simulink model "v00_0A_0E"  (R2022b)
settings: Solver=FixedStepDiscrete  StartTime=0.0  StopTime=8000  FixedStep=SampleTime  MaxStep=Contactors_StepTime_msec  RelTol=1e-3  EnableMultiTasking=on
undefined symbols (not defined in the file): A_to_mA, BalancingTempGroup, canChannel, CapacityFactor, CC_Inputs, CellSOC, ChargeState, ContactorsFlags, DiscIntNeverNeededParam, gEN_Contactors_StepTime_msec, Ion, isDynamicCurrentEn, Lithium, maxAllowedImbalance, nCells_parallel, nCells_series, nCellTempGrps, PermanentFailRecoveryTrigger, ProtectionFlags, RBal_ohm, SampleTime, sigbuilder_block, StLineEq_varA, StLineEq_varB, TempSelectForDCL, Thresholds, V_to_mV
libraries: simulink x32, spsIdealSwitchLib x21, spsBatteryLib x20, spsSeriesRLCBranchLib x20, spsVoltageMeasurementLib x20, canmsglib x4, canlib x3, dspstat3 x2, spspowerguiLib x2, spsControlledCurrentSourceLib x1, spsCurrentMeasurementLib x1
(part 2 of 7)

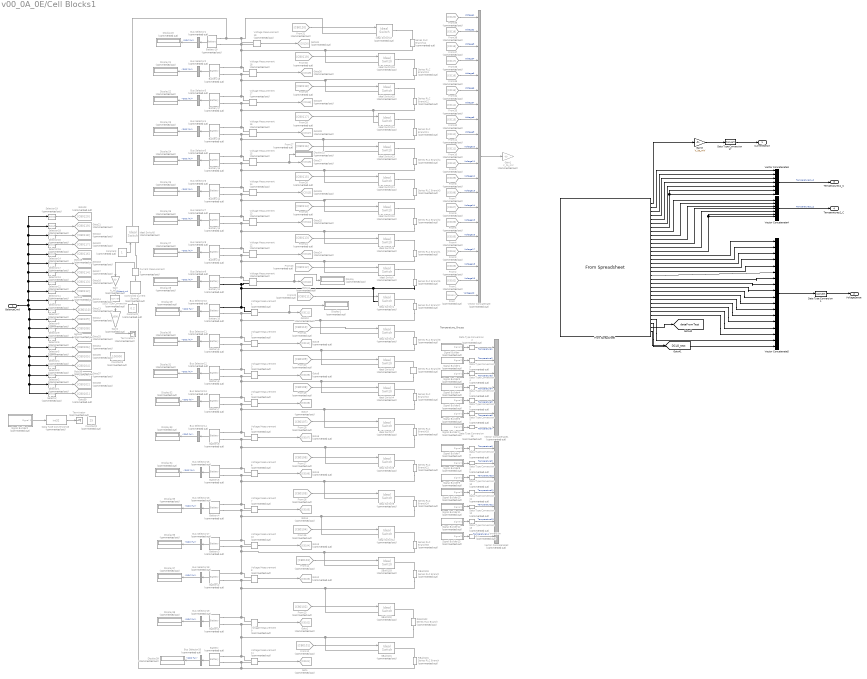
== system v00_0A_0E/Cell Blocks1 ==
  note: Temperature_Groups
  BalanceCmd : Inport
  Battery : spsBatteryLib/Battery  Commented=on  BatType=Lithium-Ion  ShowTempParam=off  ThermalPreset=no  ShowAgeParam=off  NomV=3.6  NomQ=CellCapacity_mAh  SOC=CellSOC(1)  Batt_Tr=30  PresetModel=on  MaxQ=4  MinV=2.7  FullV=4.1904  Dis_rate=1.7391  R=0.009  Normal_OP=3.6174  expZone="[3.8894     0.19652]"  current=[6.5 13 32.5]  Units=Time  Tci=20  NomT=20  T2=-30  MaxQ2=4.8  FullV2=7.1  Normal_OP2=5.655  expZone2="[6.58           1]"  Rca=0.6  ti=2000  Dp=0  Neq0=0  Tsim=1e6  Ta1=25  Qeol=5.4*0.9  Reol=0.013333*1.2  Char_age=[2.3478, 3]  Dis_age=[2.3478, 10]  N1=1500  N2=10500  N3=1000  N4=1400  Ta2=45  N5=950
  Battery1 : spsBatteryLib/Battery  Commented=on  BatType=Lithium-Ion  ShowTempParam=off  ThermalPreset=no  ShowAgeParam=off  NomV=3.6  NomQ=CellCapacity_mAh  SOC=CellSOC(2)  Batt_Tr=30  PresetModel=on  MaxQ=4  MinV=2.7  FullV=4.1904  Dis_rate=1.7391  R=0.009  Normal_OP=3.6174  expZone="[3.8894     0.19652]"  current=[6.5 13 32.5]  Units=Time  Tci=20  NomT=20  T2=-30  MaxQ2=4.8  FullV2=7.1  Normal_OP2=5.655  expZone2="[6.58           1]"  Rca=0.6  ti=2000  Dp=0  Neq0=0  Tsim=1e6  Ta1=25  Qeol=5.4*0.9  Reol=0.013333*1.2  Char_age=[2.3478, 3]  Dis_age=[2.3478, 10]  N1=1500  N2=10500  N3=1000  N4=1400  Ta2=45  N5=950
  Battery10 : spsBatteryLib/Battery  Commented=on  BatType=Lithium-Ion  ShowTempParam=off  ThermalPreset=no  ShowAgeParam=off  NomV=3.6  NomQ=CellCapacity_mAh  SOC=CellSOC(10)  Batt_Tr=30  PresetModel=on  MaxQ=4  MinV=2.7  FullV=4.1904  Dis_rate=1.7391  R=0.009  Normal_OP=3.6174  expZone="[3.8894     0.19652]"  current=[6.5 13 32.5]  Units=Time  Tci=20  NomT=20  T2=-30  MaxQ2=4.8  FullV2=7.1  Normal_OP2=5.655  expZone2="[6.58           1]"  Rca=0.6  ti=2000  Dp=0  Neq0=0  Tsim=1e6  Ta1=25  Qeol=5.4*0.9  Reol=0.013333*1.2  Char_age=[2.3478, 3]  Dis_age=[2.3478, 10]  N1=1500  N2=10500  N3=1000  N4=1400  Ta2=45  N5=950
  Battery{11..19} (9 alike) : spsBatteryLib/Battery  Commented=on  BatType=Lithium-Ion  ShowTempParam=off  ThermalPreset=no  ShowAgeParam=off  NomV=3.6  NomQ=CellCapacity_mAh  SOC=CellSOC(11)  Batt_Tr=30  PresetModel=on  MaxQ=4  MinV=2.7  FullV=4.1904  Dis_rate=1.7391  R=0.009  Normal_OP=3.6174  expZone="[3.8894     0.19652]"  current=[6.5 13 32.5]  Units=Time  Tci=20  NomT=20  T2=-30  MaxQ2=4.8  FullV2=7.1  Normal_OP2=5.655  expZone2="[6.58           1]"  Rca=0.6  ti=2000  Dp=0  Neq0=0  Tsim=1e6  Ta1=25  Qeol=5.4*0.9  Reol=0.013333*1.2  Char_age=[2.3478, 3]  Dis_age=[2.3478, 10]  N1=1500  N2=10500  N3=1000  N4=1400  Ta2=45  N5=950
  Battery2 : spsBatteryLib/Battery  Commented=on  BatType=Lithium-Ion  ShowTempParam=off  ThermalPreset=no  ShowAgeParam=off  NomV=3.6  NomQ=CellCapacity_mAh  SOC=CellSOC(3)  Batt_Tr=30  PresetModel=on  MaxQ=4  MinV=2.7  FullV=4.1904  Dis_rate=1.7391  R=0.009  Normal_OP=3.6174  expZone="[3.8894     0.19652]"  current=[6.5 13 32.5]  Units=Time  Tci=20  NomT=20  T2=-30  MaxQ2=4.8  FullV2=7.1  Normal_OP2=5.655  expZone2="[6.58           1]"  Rca=0.6  ti=2000  Dp=0  Neq0=0  Tsim=1e6  Ta1=25  Qeol=5.4*0.9  Reol=0.013333*1.2  Char_age=[2.3478, 3]  Dis_age=[2.3478, 10]  N1=1500  N2=10500  N3=1000  N4=1400  Ta2=45  N5=950
  Battery3 : spsBatteryLib/Battery  Commented=on  BatType=Lithium-Ion  ShowTempParam=off  ThermalPreset=no  ShowAgeParam=off  NomV=3.6  NomQ=CellCapacity_mAh  SOC=CellSOC(4)  Batt_Tr=30  PresetModel=on  MaxQ=4  MinV=2.7  FullV=4.1904  Dis_rate=1.7391  R=0.009  Normal_OP=3.6174  expZone="[3.8894     0.19652]"  current=[6.5 13 32.5]  Units=Time  Tci=20  NomT=20  T2=-30  MaxQ2=4.8  FullV2=7.1  Normal_OP2=5.655  expZone2="[6.58           1]"  Rca=0.6  ti=2000  Dp=0  Neq0=0  Tsim=1e6  Ta1=25  Qeol=5.4*0.9  Reol=0.013333*1.2  Char_age=[2.3478, 3]  Dis_age=[2.3478, 10]  N1=1500  N2=10500  N3=1000  N4=1400  Ta2=45  N5=950
  Battery4 : spsBatteryLib/Battery  Commented=on  BatType=Lithium-Ion  ShowTempParam=off  ThermalPreset=no  ShowAgeParam=off  NomV=3.6  NomQ=CellCapacity_mAh  SOC=CellSOC(5)  Batt_Tr=30  PresetModel=on  MaxQ=4  MinV=2.7  FullV=4.1904  Dis_rate=1.7391  R=0.009  Normal_OP=3.6174  expZone="[3.8894     0.19652]"  current=[6.5 13 32.5]  Units=Time  Tci=20  NomT=20  T2=-30  MaxQ2=4.8  FullV2=7.1  Normal_OP2=5.655  expZone2="[6.58           1]"  Rca=0.6  ti=2000  Dp=0  Neq0=0  Tsim=1e6  Ta1=25  Qeol=5.4*0.9  Reol=0.013333*1.2  Char_age=[2.3478, 3]  Dis_age=[2.3478, 10]  N1=1500  N2=10500  N3=1000  N4=1400  Ta2=45  N5=950
  Battery5 : spsBatteryLib/Battery  Commented=on  BatType=Lithium-Ion  ShowTempParam=off  ThermalPreset=no  ShowAgeParam=off  NomV=3.6  NomQ=CellCapacity_mAh  SOC=CellSOC(6)  Batt_Tr=30  PresetModel=on  MaxQ=4  MinV=2.7  FullV=4.1904  Dis_rate=1.7391  R=0.009  Normal_OP=3.6174  expZone="[3.8894     0.19652]"  current=[6.5 13 32.5]  Units=Time  Tci=20  NomT=20  T2=-30  MaxQ2=4.8  FullV2=7.1  Normal_OP2=5.655  expZone2="[6.58           1]"  Rca=0.6  ti=2000  Dp=0  Neq0=0  Tsim=1e6  Ta1=25  Qeol=5.4*0.9  Reol=0.013333*1.2  Char_age=[2.3478, 3]  Dis_age=[2.3478, 10]  N1=1500  N2=10500  N3=1000  N4=1400  Ta2=45  N5=950
  Battery6 : spsBatteryLib/Battery  Commented=on  BatType=Lithium-Ion  ShowTempParam=off  ThermalPreset=no  ShowAgeParam=off  NomV=3.6  NomQ=CellCapacity_mAh  SOC=CellSOC(7)  Batt_Tr=30  PresetModel=on  MaxQ=4  MinV=2.7  FullV=4.1904  Dis_rate=1.7391  R=0.009  Normal_OP=3.6174  expZone="[3.8894     0.19652]"  current=[6.5 13 32.5]  Units=Time  Tci=20  NomT=20  T2=-30  MaxQ2=4.8  FullV2=7.1  Normal_OP2=5.655  expZone2="[6.58           1]"  Rca=0.6  ti=2000  Dp=0  Neq0=0  Tsim=1e6  Ta1=25  Qeol=5.4*0.9  Reol=0.013333*1.2  Char_age=[2.3478, 3]  Dis_age=[2.3478, 10]  N1=1500  N2=10500  N3=1000  N4=1400  Ta2=45  N5=950
  Battery7 : spsBatteryLib/Battery  Commented=on  BatType=Lithium-Ion  ShowTempParam=off  ThermalPreset=no  ShowAgeParam=off  NomV=3.6  NomQ=CellCapacity_mAh  SOC=CellSOC(8)  Batt_Tr=30  PresetModel=on  MaxQ=4  MinV=2.7  FullV=4.1904  Dis_rate=1.7391  R=0.009  Normal_OP=3.6174  expZone="[3.8894     0.19652]"  current=[6.5 13 32.5]  Units=Time  Tci=20  NomT=20  T2=-30  MaxQ2=4.8  FullV2=7.1  Normal_OP2=5.655  expZone2="[6.58           1]"  Rca=0.6  ti=2000  Dp=0  Neq0=0  Tsim=1e6  Ta1=25  Qeol=5.4*0.9  Reol=0.013333*1.2  Char_age=[2.3478, 3]  Dis_age=[2.3478, 10]  N1=1500  N2=10500  N3=1000  N4=1400  Ta2=45  N5=950
  Battery8 : spsBatteryLib/Battery  Commented=on  BatType=Lithium-Ion  ShowTempParam=off  ThermalPreset=no  ShowAgeParam=off  NomV=3.6  NomQ=CellCapacity_mAh  SOC=CellSOC(8)  Batt_Tr=30  PresetModel=on  MaxQ=4  MinV=2.7  FullV=4.1904  Dis_rate=1.7391  R=0.009  Normal_OP=3.6174  expZone="[3.8894     0.19652]"  current=[6.5 13 32.5]  Units=Time  Tci=20  NomT=20  T2=-30  MaxQ2=4.8  FullV2=7.1  Normal_OP2=5.655  expZone2="[6.58           1]"  Rca=0.6  ti=2000  Dp=0  Neq0=0  Tsim=1e6  Ta1=25  Qeol=5.4*0.9  Reol=0.013333*1.2  Char_age=[2.3478, 3]  Dis_age=[2.3478, 10]  N1=1500  N2=10500  N3=1000  N4=1400  Ta2=45  N5=950
  Battery9 : spsBatteryLib/Battery  Commented=on  BatType=Lithium-Ion  ShowTempParam=off  ThermalPreset=no  ShowAgeParam=off  NomV=3.6  NomQ=CellCapacity_mAh  SOC=CellSOC(9)  Batt_Tr=30  PresetModel=on  MaxQ=4  MinV=2.7  FullV=4.1904  Dis_rate=1.7391  R=0.009  Normal_OP=3.6174  expZone="[3.8894     0.19652]"  current=[6.5 13 32.5]  Units=Time  Tci=20  NomT=20  T2=-30  MaxQ2=4.8  FullV2=7.1  Normal_OP2=5.655  expZone2="[6.58           1]"  Rca=0.6  ti=2000  Dp=0  Neq0=0  Tsim=1e6  Ta1=25  Qeol=5.4*0.9  Reol=0.013333*1.2  Char_age=[2.3478, 3]  Dis_age=[2.3478, 10]  N1=1500  N2=10500  N3=1000  N4=1400  Ta2=45  N5=950
  Bus Selector{1..20} (20 alike) : BusSelector  Commented=on  OutputSignals=SOC (%)
  Constant : Constant  Commented=on
  Constant1 : Constant  Commented=on  Value=0.2
  Constant2 : Constant  Commented=on  Value=25  OutDataTypeStr=int8
  Constant3 : Constant  Commented=on  Value=100000  OutDataTypeStr=int32
  Controlled Current Source1 : spsControlledCurrentSourceLib/Controlled Current Source  Commented=on  Initialize=on  Source_Type=DC  Amplitude=0.5  Phase=0  Frequency=0  Measurements=None
  Current Measurement1 : spsCurrentMeasurementLib/Current Measurement  Commented=on  PhasorSimulation=off  OutputType=Complex  PSBequivalent=0
  Data Type Conversion : DataTypeConversion  Commented=on  SaturateOnIntegerOverflow=off  RndMeth=Floor
  Data Type Conversion1 : DataTypeConversion  SaturateOnIntegerOverflow=off  RndMeth=Floor
  Data Type Conversion{2..15} (14 alike) : DataTypeConversion  Commented=on  OutDataTypeStr=int16  SaturateOnIntegerOverflow=off  RndMeth=Floor
  Data Type Conversion16 : DataTypeConversion  Commented=on  OutDataTypeStr=int32  SaturateOnIntegerOverflow=off  RndMeth=Floor
  Data Type Conversion17 : DataTypeConversion  SaturateOnIntegerOverflow=off  RndMeth=Floor
  Display{,1,15,20..39} (23 alike) : Display  Commented=on
  From : From  Commented=on  GotoTag=C0101
  From Spreadsheet : FromSpreadsheet  FileName=latchcheckcharge.xlsx
  From1 : From  Commented=on  GotoTag=C0102
  From10 : From  Commented=on  GotoTag=C0111
  From11 : From  Commented=on  GotoTag=C0112
  From12 : From  Commented=on  GotoTag=CB0101
  From13 : From  Commented=on  GotoTag=CB0102
  From14 : From  Commented=on  GotoTag=CB0103
  From15 : From  Commented=on  GotoTag=CB0104
  From16 : From  Commented=on  GotoTag=CB0105
  From17 : From  Commented=on  GotoTag=CB0106
  From18 : From  Commented=on  GotoTag=CB0107
  From19 : From  Commented=on  GotoTag=CB0108
  From2 : From  Commented=on  GotoTag=C0103
  From20 : From  Commented=on  GotoTag=CB0109
  From21 : From  Commented=on  GotoTag=CB0110
  From22 : From  Commented=on  GotoTag=CB0111
  From23 : From  Commented=on  GotoTag=CB0112
  From24 : From  Commented=on  GotoTag=CB0113
  From25 : From  Commented=on  GotoTag=CB0114
  From26 : From  Commented=on  GotoTag=CB0115
  From27 : From  Commented=on  GotoTag=CB0116
  From28 : From  Commented=on  GotoTag=CB0117
  From29 : From  Commented=on  GotoTag=CB0118
  From3 : From  Commented=on  GotoTag=C0104
  From30 : From  Commented=on  GotoTag=CB0119
  From31 : From  Commented=on  GotoTag=CB0120
  From32 : From  Commented=on  GotoTag=C0113
  From33 : From  Commented=on  GotoTag=C0114
  From34 : From  Commented=on  GotoTag=C0115
  From35 : From  Commented=on  GotoTag=C0116
  From36 : From  Commented=on  GotoTag=C0117
  From37 : From  Commented=on  GotoTag=C0118
  From38 : From  Commented=on  GotoTag=C0119
  From39 : From  Commented=on  GotoTag=C0120
  From4 : From  Commented=on  GotoTag=C0105
  From5 : From  Commented=on  GotoTag=C0106
  From6 : From  Commented=on  GotoTag=C0107
  From7 : From  Commented=on  GotoTag=C0108
  From8 : From  Commented=on  GotoTag=C0109
  From9 : From  Commented=on  GotoTag=C0110
  Gain : Gain  Commented=on  Gain=A_to_mA
  Gain1 : Gain  Commented=on  Gain=V_to_mV
  Gain2 : Gain  Commented=on  Gain=1000  OutDataTypeStr=int32
  Gain3 : Gain  Gain=V_to_mV
  Goto : Goto  Commented=on  GotoTag=C0101
  Goto1 : Goto  Commented=on  GotoTag=C0102
  Goto10 : Goto  Commented=on  GotoTag=C0111
  Goto11 : Goto  Commented=on  GotoTag=C0112
  Goto12 : Goto  Commented=on  GotoTag=CB0109
  Goto13 : Goto  Commented=on  GotoTag=CB0110
  Goto14 : Goto  Commented=on  GotoTag=CB0111
  Goto15 : Goto  Commented=on  GotoTag=CB0112
  Goto16 : Goto  Commented=on  GotoTag=CB0113
  Goto17 : Goto  Commented=on  GotoTag=CB0114
  Goto18 : Goto  Commented=on  GotoTag=CB0115
  Goto19 : Goto  Commented=on  GotoTag=CB0116
  Goto2 : Goto  Commented=on  GotoTag=C0103
  Goto20 : Goto  Commented=on  GotoTag=CB0117
  Goto21 : Goto  Commented=on  GotoTag=CB0119
  Goto22 : Goto  Commented=on  GotoTag=CB0118
  Goto23 : Goto  Commented=on  GotoTag=CB0120
  Goto24 : Goto  Commented=on  GotoTag=C0113
  Goto25 : Goto  Commented=on  GotoTag=C0114
  Goto26 : Goto  Commented=on  GotoTag=C0115
  Goto27 : Goto  Commented=on  GotoTag=C0116
  Goto28 : Goto  Commented=on  GotoTag=C0117
  Goto29 : Goto  Commented=on  GotoTag=C0118
  Goto3 : Goto  Commented=on  GotoTag=C0104
  Goto30 : Goto  Commented=on  GotoTag=C0119
  Goto31 : Goto  Commented=on  GotoTag=C0120
  Goto32 : Goto  Commented=on  GotoTag=CB0108
  Goto33 : Goto  Commented=on  GotoTag=CB0107
  Goto34 : Goto  Commented=on  GotoTag=CB0106
  Goto35 : Goto  Commented=on  GotoTag=CB0105
  Goto36 : Goto  Commented=on  GotoTag=CB0104
  Goto37 : Goto  Commented=on  GotoTag=CB0103
  Goto38 : Goto  Commented=on  GotoTag=CB0102
  Goto39 : Goto  Commented=on  GotoTag=CB0101
  Goto4 : Goto  Commented=on  GotoTag=C0105
  Goto5 : Goto  Commented=on  GotoTag=C0106
  Goto6 : Goto  Commented=on  GotoTag=C0107
  Goto7 : Goto  Commented=on  GotoTag=C0108
  Goto8 : Goto  Commented=on  GotoTag=C0109
  Goto9 : Goto  Commented=on  GotoTag=C0110
  Ideal Switch{,1..17} (18 alike) : spsIdealSwitchLib/Ideal Switch  Commented=on  Ron=0.1  Lon=0  IC=0  Rs=1e5  Cs=inf  Measurements=off
  RBal0101 : spsSeriesRLCBranchLib/Series RLC Branch  Commented=on  LConnTagsString=__new0  RConnTagsString=__new0  BranchType=R  Resistance=RBal_ohm  Inductance=0  SetiL0=off  InitialCurrent=0  Capacitance=1e-20  Setx0=off  InitialVoltage=0  Measurements=None
  RBal0102 : spsSeriesRLCBranchLib/Series RLC Branch  Commented=on  LConnTagsString=__new0  RConnTagsString=__new0  BranchType=R  Resistance=RBal_ohm  Inductance=0  SetiL0=off  InitialCurrent=0  Capacitance=1e-20  Setx0=off  InitialVoltage=0  Measurements=None
  RBal0103 : spsSeriesRLCBranchLib/Series RLC Branch  Commented=on  LConnTagsString=__new0  RConnTagsString=__new0  BranchType=R  Resistance=RBal_ohm  Inductance=0  SetiL0=off  InitialCurrent=0  Capacitance=1e-20  Setx0=off  InitialVoltage=0  Measurements=None
  SBal0101 : spsIdealSwitchLib/Ideal Switch  Commented=on  Ron=0.1  Lon=0  IC=0  Rs=1e5  Cs=inf  Measurements=off
  SBal0102 : spsIdealSwitchLib/Ideal Switch  Commented=on  Ron=0.1  Lon=0  IC=0  Rs=1e5  Cs=inf  Measurements=off
  SBal0103 : spsIdealSwitchLib/Ideal Switch  Commented=on  Ron=0.1  Lon=0  IC=0  Rs=1e5  Cs=inf  Measurements=off
  Selector : Selector  Commented=on  IndexMode=Zero-based  InputPortWidth=20  IndexOptions=Index vector (dialog)  Indices=[19]  OutputSizes=1
  Selector1 : Selector  Commented=on  IndexMode=Zero-based  InputPortWidth=20  IndexOptions=Index vector (dialog)  Indices=[18]  OutputSizes=1
  Selector10 : Selector  Commented=on  IndexMode=Zero-based  InputPortWidth=20  IndexOptions=Index vector (dialog)  Indices=[9]  OutputSizes=1
  Selector11 : Selector  Commented=on  IndexMode=Zero-based  InputPortWidth=20  IndexOptions=Index vector (dialog)  Indices=[8]  OutputSizes=1
  Selector12 : Selector  Commented=on  IndexMode=Zero-based  InputPortWidth=20  IndexOptions=Index vector (dialog)  Indices=[7]  OutputSizes=1
  Selector13 : Selector  Commented=on  IndexMode=Zero-based  InputPortWidth=20  IndexOptions=Index vector (dialog)  Indices=[6]  OutputSizes=1
  Selector14 : Selector  Commented=on  IndexMode=Zero-based  InputPortWidth=20  IndexOptions=Index vector (dialog)  Indices=[4]  OutputSizes=1
  Selector15 : Selector  Commented=on  IndexMode=Zero-based  InputPortWidth=20  IndexOptions=Index vector (dialog)  Indices=[2]  OutputSizes=1
  Selector16 : Selector  Commented=on  IndexMode=Zero-based  InputPortWidth=20  IndexOptions=Index vector (dialog)  Indices=[3]  OutputSizes=1
  Selector17 : Selector  Commented=on  IndexMode=Zero-based  InputPortWidth=20  IndexOptions=Index vector (dialog)  Indices=[5]  OutputSizes=1
  Selector18 : Selector  Commented=on  IndexMode=Zero-based  InputPortWidth=20  IndexOptions=Index vector (dialog)  Indices=[1]  OutputSizes=1
  Selector19 : Selector  Commented=on  IndexMode=Zero-based  InputPortWidth=20  IndexOptions=Index vector (dialog)  Indices=[0]  OutputSizes=1
  Selector2 : Selector  Commented=on  IndexMode=Zero-based  InputPortWidth=20  IndexOptions=Index vector (dialog)  Indices=[17]  OutputSizes=1
  Selector3 : Selector  Commented=on  IndexMode=Zero-based  InputPortWidth=20  IndexOptions=Index vector (dialog)  Indices=[16]  OutputSizes=1
  Selector4 : Selector  Commented=on  IndexMode=Zero-based  InputPortWidth=20  IndexOptions=Index vector (dialog)  Indices=[15]  OutputSizes=1
  Selector5 : Selector  Commented=on  IndexMode=Zero-based  InputPortWidth=20  IndexOptions=Index vector (dialog)  Indices=[14]  OutputSizes=1
  Selector6 : Selector  Commented=on  IndexMode=Zero-based  InputPortWidth=20  IndexOptions=Index vector (dialog)  Indices=[13]  OutputSizes=1
  Selector7 : Selector  Commented=on  IndexMode=Zero-based  InputPortWidth=20  IndexOptions=Index vector (dialog)  Indices=[10]  OutputSizes=1
  Selector8 : Selector  Commented=on  IndexMode=Zero-based  InputPortWidth=20  IndexOptions=Index vector (dialog)  Indices=[11]  OutputSizes=1
  Selector9 : Selector  Commented=on  IndexMode=Zero-based  InputPortWidth=20  IndexOptions=Index vector (dialog)  Indices=[12]  OutputSizes=1
  Series RLC Branch{1..5,7..14,18,21,24,33} (17 alike) : spsSeriesRLCBranchLib/Series RLC Branch  Commented=on  LConnTagsString=__new0  RConnTagsString=__new0  BranchType=R  Resistance=RBal_ohm  Inductance=0  SetiL0=off  InitialCurrent=0  Capacitance=1e-20  Setx0=off  InitialVoltage=0  Measurements=None
  Signal Builder : Subsystem  Tag=STV Subsys  Commented=on  LoadFcn=sigbuilder_block('load');  StartFcn=sigbuilder_block('start');  StopFcn=sigbuilder_block('stop');  ClipboardFcn=sigbuilder_block('clipboard');  mask(Sigbuilder block){tuvar=[0:10]}
      mask help: Simulink:masks:SigbuilderBlock_MD
      mask init:
      | if ~strcmp(get_param(bdroot(gcbh),'SimulationStatus'),'stopped') tuvar = sigbuilder_block('maskInit'); end
      settings: CopyFcn=sigbuilder_block('copy');  DeleteFcn=sigbuilder_block('delete');  ModelCloseFcn=sigbuilder_block('modelClose');  PreSaveFcn=sigbuilder_block('preSave');  PauseFcn=sigbuilder_block('pause');  ContinueFcn=sigbuilder_block('continue');  NameChangeFcn=sigbuilder_block('namechange');  OpenFcn=sigbuilder_block('open',[5.4 30 1141.2 522.6 ]);  CloseFcn=sigbuilder_block('close');
      mask Display: plot(0, 0, 100, 100,[2, 2, 32, 32, 2], [68, 8, 8, 68, 68],[32, 2], [38, 38], [32, 19, 2],[53, 60, 44], [32, 17, 17, 2],[16, 16, 31, 31]);txt = getActiveGroup(gcbh);text(2, 100, txt,'verticalAlignment', 'top');
  Signal Builder1 : Subsystem  Tag=STV Subsys  Commented=on  LoadFcn=sigbuilder_block('load');  StartFcn=sigbuilder_block('start');  StopFcn=sigbuilder_block('stop');  ClipboardFcn=sigbuilder_block('clipboard');  mask(Sigbuilder block){tuvar=[0:10]}
      mask help: Simulink:masks:SigbuilderBlock_MD
      mask init:
      | if ~strcmp(get_param(bdroot(gcbh),'SimulationStatus'),'stopped') tuvar = sigbuilder_block('maskInit'); end
      settings: CopyFcn=sigbuilder_block('copy');  DeleteFcn=sigbuilder_block('delete');  ModelCloseFcn=sigbuilder_block('modelClose');  PreSaveFcn=sigbuilder_block('preSave');  PauseFcn=sigbuilder_block('pause');  ContinueFcn=sigbuilder_block('continue');  NameChangeFcn=sigbuilder_block('namechange');  OpenFcn=sigbuilder_block('open',[5.4 30 1141.2 522.6 ]);  CloseFcn=sigbuilder_block('close');
      mask Display: plot(0, 0, 100, 100,[2, 2, 32, 32, 2], [68, 8, 8, 68, 68],[32, 2], [38, 38], [32, 19, 2],[53, 60, 44], [32, 17, 17, 2],[16, 16, 31, 31]);txt = getActiveGroup(gcbh);text(2, 100, txt,'verticalAlignment', 'top');
  Signal Builder10 : Subsystem  Tag=STV Subsys  Commented=on  LoadFcn=sigbuilder_block('load');  StartFcn=sigbuilder_block('start');  StopFcn=sigbuilder_block('stop');  ClipboardFcn=sigbuilder_block('clipboard');  mask(Sigbuilder block){tuvar=[0:10]}
      mask help: Simulink:masks:SigbuilderBlock_MD
      mask init:
      | if ~strcmp(get_param(bdroot(gcbh),'SimulationStatus'),'stopped') tuvar = sigbuilder_block('maskInit'); end
      settings: CopyFcn=sigbuilder_block('copy');  DeleteFcn=sigbuilder_block('delete');  ModelCloseFcn=sigbuilder_block('modelClose');  PreSaveFcn=sigbuilder_block('preSave');  PauseFcn=sigbuilder_block('pause');  ContinueFcn=sigbuilder_block('continue');  NameChangeFcn=sigbuilder_block('namechange');  OpenFcn=sigbuilder_block('open',[0 30 1152 561.6 ]);  CloseFcn=sigbuilder_block('close');
      mask Display: plot(0, 0, 100, 100,[2, 2, 32, 32, 2], [68, 8, 8, 68, 68],[32, 2], [38, 38], [32, 19, 2],[53, 60, 44], [32, 17, 17, 2],[16, 16, 31, 31]);txt = getActiveGroup(gcbh);text(2, 100, txt,'verticalAlignment', 'top');
  Signal Builder11 : Subsystem  Tag=STV Subsys  Commented=on  LoadFcn=sigbuilder_block('load');  StartFcn=sigbuilder_block('start');  StopFcn=sigbuilder_block('stop');  ClipboardFcn=sigbuilder_block('clipboard');  mask(Sigbuilder block){tuvar=[0:10]}
      mask help: Simulink:masks:SigbuilderBlock_MD
      mask init:
      | if ~strcmp(get_param(bdroot(gcbh),'SimulationStatus'),'stopped') tuvar = sigbuilder_block('maskInit'); end
      settings: CopyFcn=sigbuilder_block('copy');  DeleteFcn=sigbuilder_block('delete');  ModelCloseFcn=sigbuilder_block('modelClose');  PreSaveFcn=sigbuilder_block('preSave');  PauseFcn=sigbuilder_block('pause');  ContinueFcn=sigbuilder_block('continue');  NameChangeFcn=sigbuilder_block('namechange');  OpenFcn=sigbuilder_block('open',[0 30 1152 561.6 ]);  CloseFcn=sigbuilder_block('close');
      mask Display: plot(0, 0, 100, 100,[2, 2, 32, 32, 2], [68, 8, 8, 68, 68],[32, 2], [38, 38], [32, 19, 2],[53, 60, 44], [32, 17, 17, 2],[16, 16, 31, 31]);txt = getActiveGroup(gcbh);text(2, 100, txt,'verticalAlignment', 'top');
  Signal Builder12 : Subsystem  Tag=STV Subsys  Commented=on  LoadFcn=sigbuilder_block('load');  StartFcn=sigbuilder_block('start');  StopFcn=sigbuilder_block('stop');  ClipboardFcn=sigbuilder_block('clipboard');  mask(Sigbuilder block){tuvar=[0:10]}
      mask help: Simulink:masks:SigbuilderBlock_MD
      mask init:
      | if ~strcmp(get_param(bdroot(gcbh),'SimulationStatus'),'stopped') tuvar = sigbuilder_block('maskInit'); end
      settings: CopyFcn=sigbuilder_block('copy');  DeleteFcn=sigbuilder_block('delete');  ModelCloseFcn=sigbuilder_block('modelClose');  PreSaveFcn=sigbuilder_block('preSave');  PauseFcn=sigbuilder_block('pause');  ContinueFcn=sigbuilder_block('continue');  NameChangeFcn=sigbuilder_block('namechange');  OpenFcn=sigbuilder_block('open',[0 30 1152 561.6 ]);  CloseFcn=sigbuilder_block('close');
      mask Display: plot(0, 0, 100, 100,[2, 2, 32, 32, 2], [68, 8, 8, 68, 68],[32, 2], [38, 38], [32, 19, 2],[53, 60, 44], [32, 17, 17, 2],[16, 16, 31, 31]);txt = getActiveGroup(gcbh);text(2, 100, txt,'verticalAlignment', 'top');
  Signal Builder13 : Subsystem  Tag=STV Subsys  Commented=on  LoadFcn=sigbuilder_block('load');  StartFcn=sigbuilder_block('start');  StopFcn=sigbuilder_block('stop');  ClipboardFcn=sigbuilder_block('clipboard');  mask(Sigbuilder block){tuvar=[0:10]}
      mask help: Simulink:masks:SigbuilderBlock_MD
      mask init:
      | if ~strcmp(get_param(bdroot(gcbh),'SimulationStatus'),'stopped') tuvar = sigbuilder_block('maskInit'); end
      settings: CopyFcn=sigbuilder_block('copy');  DeleteFcn=sigbuilder_block('delete');  ModelCloseFcn=sigbuilder_block('modelClose');  PreSaveFcn=sigbuilder_block('preSave');  PauseFcn=sigbuilder_block('pause');  ContinueFcn=sigbuilder_block('continue');  NameChangeFcn=sigbuilder_block('namechange');  OpenFcn=sigbuilder_block('open',[0 30 1152 561.6 ]);  CloseFcn=sigbuilder_block('close');
      mask Display: plot(0, 0, 100, 100,[2, 2, 32, 32, 2], [68, 8, 8, 68, 68],[32, 2], [38, 38], [32, 19, 2],[53, 60, 44], [32, 17, 17, 2],[16, 16, 31, 31]);txt = getActiveGroup(gcbh);text(2, 100, txt,'verticalAlignment', 'top');
  Signal Builder14 : Subsystem  Tag=STV Subsys  Commented=on  LoadFcn=sigbuilder_block('load');  StartFcn=sigbuilder_block('start');  StopFcn=sigbuilder_block('stop');  ClipboardFcn=sigbuilder_block('clipboard');  mask(Sigbuilder block){tuvar=[0:10]}
      mask help: Simulink:masks:SigbuilderBlock_MD
      mask init:
      | if ~strcmp(get_param(bdroot(gcbh),'SimulationStatus'),'stopped') tuvar = sigbuilder_block('maskInit'); end
      settings: CopyFcn=sigbuilder_block('copy');  DeleteFcn=sigbuilder_block('delete');  ModelCloseFcn=sigbuilder_block('modelClose');  PreSaveFcn=sigbuilder_block('preSave');  PauseFcn=sigbuilder_block('pause');  ContinueFcn=sigbuilder_block('continue');  NameChangeFcn=sigbuilder_block('namechange');  OpenFcn=sigbuilder_block('open',[5.4 30 1141.2 522.6 ]);  CloseFcn=sigbuilder_block('close');
      mask Display: plot(0, 0, 100, 100,[2, 2, 32, 32, 2], [68, 8, 8, 68, 68],[32, 2], [38, 38], [32, 19, 2],[53, 60, 44], [32, 17, 17, 2],[16, 16, 31, 31]);txt = getActiveGroup(gcbh);text(2, 100, txt,'verticalAlignment', 'top');
  Signal Builder2 : Subsystem  Tag=STV Subsys  Commented=on  LoadFcn=sigbuilder_block('load');  StartFcn=sigbuilder_block('start');  StopFcn=sigbuilder_block('stop');  ClipboardFcn=sigbuilder_block('clipboard');  mask(Sigbuilder block){tuvar=[0:10]}
      mask help: Simulink:masks:SigbuilderBlock_MD
      mask init:
      | if ~strcmp(get_param(bdroot(gcbh),'SimulationStatus'),'stopped') tuvar = sigbuilder_block('maskInit'); end
      settings: CopyFcn=sigbuilder_block('copy');  DeleteFcn=sigbuilder_block('delete');  ModelCloseFcn=sigbuilder_block('modelClose');  PreSaveFcn=sigbuilder_block('preSave');  PauseFcn=sigbuilder_block('pause');  ContinueFcn=sigbuilder_block('continue');  NameChangeFcn=sigbuilder_block('namechange');  OpenFcn=sigbuilder_block('open',[0 30 1152 561.6 ]);  CloseFcn=sigbuilder_block('close');
      mask Display: plot(0, 0, 100, 100,[2, 2, 32, 32, 2], [68, 8, 8, 68, 68],[32, 2], [38, 38], [32, 19, 2],[53, 60, 44], [32, 17, 17, 2],[16, 16, 31, 31]);txt = getActiveGroup(gcbh);text(2, 100, txt,'verticalAlignment', 'top');
  Signal Builder3 : Subsystem  Tag=STV Subsys  Commented=on  LoadFcn=sigbuilder_block('load');  StartFcn=sigbuilder_block('start');  StopFcn=sigbuilder_block('stop');  ClipboardFcn=sigbuilder_block('clipboard');  mask(Sigbuilder block){tuvar=[0:10]}
      mask help: Simulink:masks:SigbuilderBlock_MD
      mask init:
      | if ~strcmp(get_param(bdroot(gcbh),'SimulationStatus'),'stopped') tuvar = sigbuilder_block('maskInit'); end
      settings: CopyFcn=sigbuilder_block('copy');  DeleteFcn=sigbuilder_block('delete');  ModelCloseFcn=sigbuilder_block('modelClose');  PreSaveFcn=sigbuilder_block('preSave');  PauseFcn=sigbuilder_block('pause');  ContinueFcn=sigbuilder_block('continue');  NameChangeFcn=sigbuilder_block('namechange');  OpenFcn=sigbuilder_block('open',[5.4 30 1141.2 522.6 ]);  CloseFcn=sigbuilder_block('close');
      mask Display: plot(0, 0, 100, 100,[2, 2, 32, 32, 2], [68, 8, 8, 68, 68],[32, 2], [38, 38], [32, 19, 2],[53, 60, 44], [32, 17, 17, 2],[16, 16, 31, 31]);txt = getActiveGroup(gcbh);text(2, 100, txt,'verticalAlignment', 'top');
  Signal Builder4 : Subsystem  Tag=STV Subsys  Commented=on  LoadFcn=sigbuilder_block('load');  StartFcn=sigbuilder_block('start');  StopFcn=sigbuilder_block('stop');  ClipboardFcn=sigbuilder_block('clipboard');  mask(Sigbuilder block){tuvar=[0:10]}
      mask help: Simulink:masks:SigbuilderBlock_MD
      mask init:
      | if ~strcmp(get_param(bdroot(gcbh),'SimulationStatus'),'stopped') tuvar = sigbuilder_block('maskInit'); end
      settings: CopyFcn=sigbuilder_block('copy');  DeleteFcn=sigbuilder_block('delete');  ModelCloseFcn=sigbuilder_block('modelClose');  PreSaveFcn=sigbuilder_block('preSave');  PauseFcn=sigbuilder_block('pause');  ContinueFcn=sigbuilder_block('continue');  NameChangeFcn=sigbuilder_block('namechange');  OpenFcn=sigbuilder_block('open',[0 30 1152 561.6 ]);  CloseFcn=sigbuilder_block('close');
      mask Display: plot(0, 0, 100, 100,[2, 2, 32, 32, 2], [68, 8, 8, 68, 68],[32, 2], [38, 38], [32, 19, 2],[53, 60, 44], [32, 17, 17, 2],[16, 16, 31, 31]);txt = getActiveGroup(gcbh);text(2, 100, txt,'verticalAlignment', 'top');
  Signal Builder5 : Subsystem  Tag=STV Subsys  Commented=on  LoadFcn=sigbuilder_block('load');  StartFcn=sigbuilder_block('start');  StopFcn=sigbuilder_block('stop');  ClipboardFcn=sigbuilder_block('clipboard');  mask(Sigbuilder block){tuvar=[0:10]}
      mask help: Simulink:masks:SigbuilderBlock_MD
      mask init:
      | if ~strcmp(get_param(bdroot(gcbh),'SimulationStatus'),'stopped') tuvar = sigbuilder_block('maskInit'); end
      settings: CopyFcn=sigbuilder_block('copy');  DeleteFcn=sigbuilder_block('delete');  ModelCloseFcn=sigbuilder_block('modelClose');  PreSaveFcn=sigbuilder_block('preSave');  PauseFcn=sigbuilder_block('pause');  ContinueFcn=sigbuilder_block('continue');  NameChangeFcn=sigbuilder_block('namechange');  OpenFcn=sigbuilder_block('open',[5.4 30 1141.2 522.6 ]);  CloseFcn=sigbuilder_block('close');
      mask Display: plot(0, 0, 100, 100,[2, 2, 32, 32, 2], [68, 8, 8, 68, 68],[32, 2], [38, 38], [32, 19, 2],[53, 60, 44], [32, 17, 17, 2],[16, 16, 31, 31]);txt = getActiveGroup(gcbh);text(2, 100, txt,'verticalAlignment', 'top');
  Signal Builder6 : Subsystem  Tag=STV Subsys  Commented=on  LoadFcn=sigbuilder_block('load');  StartFcn=sigbuilder_block('start');  StopFcn=sigbuilder_block('stop');  ClipboardFcn=sigbuilder_block('clipboard');  mask(Sigbuilder block){tuvar=[0:10]}
      mask help: Simulink:masks:SigbuilderBlock_MD
      mask init:
      | if ~strcmp(get_param(bdroot(gcbh),'SimulationStatus'),'stopped') tuvar = sigbuilder_block('maskInit'); end
      settings: CopyFcn=sigbuilder_block('copy');  DeleteFcn=sigbuilder_block('delete');  ModelCloseFcn=sigbuilder_block('modelClose');  PreSaveFcn=sigbuilder_block('preSave');  PauseFcn=sigbuilder_block('pause');  ContinueFcn=sigbuilder_block('continue');  NameChangeFcn=sigbuilder_block('namechange');  OpenFcn=sigbuilder_block('open',[5.4 30 1141.2 522.6 ]);  CloseFcn=sigbuilder_block('close');
      mask Display: plot(0, 0, 100, 100,[2, 2, 32, 32, 2], [68, 8, 8, 68, 68],[32, 2], [38, 38], [32, 19, 2],[53, 60, 44], [32, 17, 17, 2],[16, 16, 31, 31]);txt = getActiveGroup(gcbh);text(2, 100, txt,'verticalAlignment', 'top');
  Signal Builder7 : Subsystem  Tag=STV Subsys  Commented=on  LoadFcn=sigbuilder_block('load');  StartFcn=sigbuilder_block('start');  StopFcn=sigbuilder_block('stop');  ClipboardFcn=sigbuilder_block('clipboard');  mask(Sigbuilder block){tuvar=[0:10]}
      mask help: Simulink:masks:SigbuilderBlock_MD
      mask init:
      | if ~strcmp(get_param(bdroot(gcbh),'SimulationStatus'),'stopped') tuvar = sigbuilder_block('maskInit'); end
      settings: CopyFcn=sigbuilder_block('copy');  DeleteFcn=sigbuilder_block('delete');  ModelCloseFcn=sigbuilder_block('modelClose');  PreSaveFcn=sigbuilder_block('preSave');  PauseFcn=sigbuilder_block('pause');  ContinueFcn=sigbuilder_block('continue');  NameChangeFcn=sigbuilder_block('namechange');  OpenFcn=sigbuilder_block('open',[5.4 30 1141.2 522.6 ]);  CloseFcn=sigbuilder_block('close');
      mask Display: plot(0, 0, 100, 100,[2, 2, 32, 32, 2], [68, 8, 8, 68, 68],[32, 2], [38, 38], [32, 19, 2],[53, 60, 44], [32, 17, 17, 2],[16, 16, 31, 31]);txt = getActiveGroup(gcbh);text(2, 100, txt,'verticalAlignment', 'top');
  Signal Builder8 : Subsystem  Tag=STV Subsys  Commented=on  LoadFcn=sigbuilder_block('load');  StartFcn=sigbuilder_block('start');  StopFcn=sigbuilder_block('stop');  ClipboardFcn=sigbuilder_block('clipboard');  mask(Sigbuilder block){tuvar=[0:10]}
      mask help: Simulink:masks:SigbuilderBlock_MD
      mask init:
      | if ~strcmp(get_param(bdroot(gcbh),'SimulationStatus'),'stopped') tuvar = sigbuilder_block('maskInit'); end
      settings: CopyFcn=sigbuilder_block('copy');  DeleteFcn=sigbuilder_block('delete');  ModelCloseFcn=sigbuilder_block('modelClose');  PreSaveFcn=sigbuilder_block('preSave');  PauseFcn=sigbuilder_block('pause');  ContinueFcn=sigbuilder_block('continue');  NameChangeFcn=sigbuilder_block('namechange');  OpenFcn=sigbuilder_block('open',[5.4 30 1141.2 522.6 ]);  CloseFcn=sigbuilder_block('close');
      mask Display: plot(0, 0, 100, 100,[2, 2, 32, 32, 2], [68, 8, 8, 68, 68],[32, 2], [38, 38], [32, 19, 2],[53, 60, 44], [32, 17, 17, 2],[16, 16, 31, 31]);txt = getActiveGroup(gcbh);text(2, 100, txt,'verticalAlignment', 'top');
  Signal Builder9 : Subsystem  Tag=STV Subsys  Commented=on  LoadFcn=sigbuilder_block('load');  StartFcn=sigbuilder_block('start');  StopFcn=sigbuilder_block('stop');  ClipboardFcn=sigbuilder_block('clipboard');  mask(Sigbuilder block){tuvar=[0:10]}
      mask help: Simulink:masks:SigbuilderBlock_MD
      mask init:
      | if ~strcmp(get_param(bdroot(gcbh),'SimulationStatus'),'stopped') tuvar = sigbuilder_block('maskInit'); end
      settings: CopyFcn=sigbuilder_block('copy');  DeleteFcn=sigbuilder_block('delete');  ModelCloseFcn=sigbuilder_block('modelClose');  PreSaveFcn=sigbuilder_block('preSave');  PauseFcn=sigbuilder_block('pause');  ContinueFcn=sigbuilder_block('continue');  NameChangeFcn=sigbuilder_block('namechange');  OpenFcn=sigbuilder_block('open',[0 30 1152 561.6 ]);  CloseFcn=sigbuilder_block('close');
      mask Display: plot(0, 0, 100, 100,[2, 2, 32, 32, 2], [68, 8, 8, 68, 68],[32, 2], [38, 38], [32, 19, 2],[53, 60, 44], [32, 17, 17, 2],[16, 16, 31, 31]);txt = getActiveGroup(gcbh);text(2, 100, txt,'verticalAlignment', 'top');
  Terminator : Terminator  Commented=on
  Terminator1 : Terminator  Commented=on
  Vector Concatenate : Concatenate  Commented=on  NumInputs=20
  Vector Concatenate1 : Concatenate  Commented=on  NumInputs=7
  Vector Concatenate2 : Concatenate  Commented=on  NumInputs=7
  Vector Concatenate3 : Concatenate  NumInputs=7
  Vector Concatenate4 : Concatenate  NumInputs=7
  Vector Concatenate5 : Concatenate  NumInputs=18
  Voltage Measurement{,1..19} (20 alike) : spsVoltageMeasurementLib/Voltage Measurement  Commented=on  PhasorSimulation=off  OutputType=Complex  PSBequivalent=0
  CurrentSense : Outport
  VoltageSense : Outport  Port=2
  Temperatures1_C : Outport  Port=3
  Temperatures2_C : Outport  Port=4
  tag scope: DCLO_test=global, dataFromTest=global
  wires:
  From21/1 -> Ideal Switch2/1
  Voltage Measurement9/1 -> Goto1/1
  Voltage Measurement2/1 -> Goto9/1
  Voltage Measurement6/1 -> Goto5/1
  Voltage Measurement7/1 -> Goto4/1
  From20/1 -> Ideal Switch3/1
  From18/1 -> Ideal Switch7/1
  From13/1 -> SBal0102/1
  Voltage Measurement/1 -> Display/1, Goto11/1
  From22/1 -> Ideal Switch1/1
  From12/1 -> SBal0101/1
  Voltage Measurement8/1 -> Goto2/1
  Voltage Measurement5/1 -> Goto6/1
  From19/1 -> Ideal Switch4/1
  Voltage Measurement10/1 -> Goto3/1
  Constant/1 -> Ideal Switch5/1
  From14/1 -> SBal0103/1
  Voltage Measurement11/1 -> Goto/1
  Voltage Measurement3/1 -> Goto8/1
  From15/1 -> Ideal Switch12/1
  From23/1 -> Ideal Switch/1
  From17/1 -> Ideal Switch8/1
  Voltage Measurement4/1 -> Goto7/1
  From3/1 -> Vector Concatenate/17  "Voltage17"
  From11/1 -> Vector Concatenate/9  "Voltage9"
  From10/1 -> Vector Concatenate/10  "Voltage10"
  From9/1 -> Vector Concatenate/11  "Voltage11"
  From8/1 -> Vector Concatenate/12  "Voltage12"
  From7/1 -> Vector Concatenate/13  "Voltage13"
  From6/1 -> Vector Concatenate/14  "Voltage14"
  From5/1 -> Vector Concatenate/15  "Voltage15"
  From4/1 -> Vector Concatenate/16  "Voltage16"
  From16/1 -> Ideal Switch9/1
  Voltage Measurement12/1 -> Goto24/1
  From24/1 -> Ideal Switch6/1
  Voltage Measurement13/1 -> Goto25/1
  From25/1 -> Ideal Switch10/1
  Voltage Measurement14/1 -> Goto26/1
  From26/1 -> Ideal Switch11/1
  Voltage Measurement15/1 -> Display15/1, Goto27/1
  From27/1 -> Ideal Switch13/1
  Voltage Measurement16/1 -> Goto28/1
  From28/1 -> Ideal Switch14/1
  Voltage Measurement17/1 -> Goto29/1
  From29/1 -> Ideal Switch15/1
  Voltage Measurement18/1 -> Goto30/1
  From30/1 -> Ideal Switch16/1
  Voltage Measurement19/1 -> Goto31/1
  From31/1 -> Ideal Switch17/1
  From39/1 -> Vector Concatenate/1  "Voltage1"
  From38/1 -> Vector Concatenate/2  "Voltage2"
  From37/1 -> Vector Concatenate/3  "Voltage3"
  From36/1 -> Vector Concatenate/4  "Voltage4"
  From35/1 -> Vector Concatenate/5  "Voltage5"
  From34/1 -> Vector Concatenate/6  "Voltage6"
  From33/1 -> Vector Concatenate/7  "Voltage7"
  From32/1 -> Vector Concatenate/8  "Voltage8"
  Selector19/1 -> Goto23/1
  Selector18/1 -> Goto21/1
  Selector15/1 -> Goto22/1
  Selector16/1 -> Goto20/1
  Selector14/1 -> Goto19/1
  Selector17/1 -> Goto18/1
  Selector13/1 -> Goto17/1
  Selector12/1 -> Goto16/1
  Selector11/1 -> Goto15/1
  Selector10/1 -> Goto14/1
  Selector7/1 -> Goto13/1
  Selector8/1 -> Goto12/1
  Selector9/1 -> Goto32/1
  Selector6/1 -> Goto33/1
  Selector5/1 -> Goto34/1
  Selector4/1 -> Goto35/1
  Selector3/1 -> Goto36/1
  Selector2/1 -> Goto37/1
  Selector1/1 -> Goto38/1
  Selector/1 -> Goto39/1
  Bus Selector2/1 -> Display21/1  "<SOC (%)>"
  Battery18/1 -> Bus Selector2/1
  Battery17/1 -> Bus Selector3/1
  Bus Selector3/1 -> Display22/1  "<SOC (%)>"
  Bus Selector4/1 -> Display23/1  "<SOC (%)>"
  Battery16/1 -> Bus Selector4/1
  Battery15/1 -> Bus Selector5/1
  Bus Selector5/1 -> Display24/1  "<SOC (%)>"
  Bus Selector6/1 -> Display25/1  "<SOC (%)>"
  Battery14/1 -> Bus Selector6/1
  Battery13/1 -> Bus Selector7/1
  Bus Selector7/1 -> Display26/1  "<SOC (%)>"
  Bus Selector8/1 -> Display27/1  "<SOC (%)>"
  Battery12/1 -> Bus Selector8/1
  Battery11/1 -> Bus Selector9/1
  Bus Selector9/1 -> Display28/1  "<SOC (%)>"
  Bus Selector10/1 -> Display29/1  "<SOC (%)>"
  Battery10/1 -> Bus Selector10/1
  Battery9/1 -> Bus Selector11/1
  Bus Selector11/1 -> Display30/1  "<SOC (%)>"
  Bus Selector12/1 -> Display31/1  "<SOC (%)>"
  Battery8/1 -> Bus Selector12/1
  Battery7/1 -> Bus Selector13/1
  Bus Selector13/1 -> Display32/1  "<SOC (%)>"
  Bus Selector14/1 -> Display33/1  "<SOC (%)>"
  Battery6/1 -> Bus Selector14/1
  Bus Selector15/1 -> Display34/1  "<SOC (%)>"
  Battery5/1 -> Bus Selector15/1
  Bus Selector16/1 -> Display35/1  "<SOC (%)>"
  Battery4/1 -> Bus Selector16/1
  Battery3/1 -> Bus Selector17/1
  Bus Selector17/1 -> Display36/1  "<SOC (%)>"
  Bus Selector18/1 -> Display37/1  "<SOC (%)>"
  Battery2/1 -> Bus Selector18/1
  Bus Selector19/1 -> Display38/1  "<SOC (%)>"
  Bus Selector20/1 -> Display39/1  "<SOC (%)>"
  Battery/1 -> Bus Selector20/1
  Constant1/1 -> Controlled Current Source1/1
  BalanceCmd/1 -> Selector6/1, Selector2/1, Selector1/1, Selector/1, Selector3/1, Selector4/1, Selector5/1, Selector9/1, Selector8/1, Selector7/1, Selector10/1, Selector11/1, Selector12/1, Selector13/1, Selector17/1, Selector14/1, Selector16/1, Selector15/1, Selector18/1, Selector19/1
  Current Measurement1/1 -> Gain/1
  Gain/1 -> Data Type Conversion/1  "Current_mA"
  Data Type Conversion1/1 -> VoltageSense/1
  From2/1 -> Vector Concatenate/18  "Voltage18"
  From1/1 -> Vector Concatenate/19  "Voltage19"
  From/1 -> Vector Concatenate/20  "Voltage20"
  Data Type Conversion12/1 -> Vector Concatenate2/5  "Temperature12"
  Data Type Conversion3/1 -> Vector Concatenate1/2  "Temperature2"
  Signal Builder/1(Signal 1) -> Data Type Conversion2/1
  Data Type Conversion10/1 -> Vector Concatenate2/3  "Temperature10"
  Data Type Conversion4/1 -> Vector Concatenate1/3  "Temperature3"
  Signal Builder6/1(Signal 1) -> Data Type Conversion7/1
  Data Type Conversion5/1 -> Vector Concatenate1/4  "Temperature4"
  Data Type Conversion13/1 -> Vector Concatenate2/6  "Temperature13"
  Data Type Conversion11/1 -> Vector Concatenate2/4  "Temperature11"
  Signal Builder5/1(Signal 1) -> Data Type Conversion6/1
  Battery1/1 -> Bus Selector19/1
  Voltage Measurement1/1 -> Display1/1, Goto10/1
  Data Type Conversion/1 -> Gain2/1
  Data Type Conversion2/1 -> Vector Concatenate1/1  "Temperature1"
  Signal Builder1/1(Signal 1) -> Data Type Conversion3/1
  Signal Builder3/1(Signal 1) -> Data Type Conversion4/1
  Signal Builder4/1(Signal 1) -> Data Type Conversion5/1
  Signal Builder7/1(Signal 1) -> Data Type Conversion8/1
  Signal Builder8/1(Signal 1) -> Data Type Conversion9/1
  Signal Builder9/1(Signal 1) -> Data Type Conversion10/1
  Signal Builder10/1(Signal 1) -> Data Type Conversion11/1
  Data Type Conversion7/1 -> Vector Concatenate1/6  "Temperature6"
  Data Type Conversion6/1 -> Vector Concatenate1/5  "Temperature5"
  Data Type Conversion8/1 -> Vector Concatenate2/1  "Temperature8"
  Data Type Conversion9/1 -> Vector Concatenate2/2  "Temperature9"
  Data Type Conversion14/1 -> Vector Concatenate2/7  "Temperature14"
  Signal Builder14/1(Signal 1) -> Data Type Conversion15/1
  Data Type Conversion15/1 -> Vector Concatenate1/7  "Temperature7"
  Signal Builder11/1(Signal 1) -> Data Type Conversion12/1
  Signal Builder12/1(Signal 1) -> Data Type Conversion13/1
  Signal Builder13/1(Signal 1) -> Data Type Conversion14/1
  Signal Builder2/1(Signal 1) -> Data Type Conversion16/1
  Data Type Conversion16/1 -> Terminator/1
  Gain2/1 -> Terminator1/1
  Battery19/1 -> Bus Selector1/1
  Bus Selector1/1 -> Display20/1  "<SOC (%)>"
  From Spreadsheet/1 -> Gain3/1
  Gain3/1 -> Data Type Conversion17/1
  From Spreadsheet/2 -> Vector Concatenate3/1
  From Spreadsheet/3 -> Vector Concatenate3/2
  From Spreadsheet/4 -> Vector Concatenate3/3
  From Spreadsheet/5 -> Vector Concatenate3/4
  From Spreadsheet/6 -> Vector Concatenate3/5
  From Spreadsheet/7 -> Vector Concatenate3/7, Vector Concatenate3/6
  From Spreadsheet/8 -> Vector Concatenate4/1
  From Spreadsheet/9 -> Vector Concatenate4/2
  From Spreadsheet/10 -> Vector Concatenate4/3
  From Spreadsheet/11 -> Vector Concatenate4/4
  From Spreadsheet/12 -> Vector Concatenate4/5
  From Spreadsheet/13 -> Vector Concatenate4/7, Vector Concatenate4/6
  From Spreadsheet/15 -> Vector Concatenate5/2
  From Spreadsheet/14 -> Vector Concatenate5/1
  From Spreadsheet/16 -> Vector Concatenate5/3
  From Spreadsheet/17 -> Vector Concatenate5/4
  From Spreadsheet/18 -> Vector Concatenate5/5
  From Spreadsheet/19 -> Vector Concatenate5/6
  From Spreadsheet/20 -> Vector Concatenate5/7
  From Spreadsheet/21 -> Vector Concatenate5/8
  From Spreadsheet/22 -> Vector Concatenate5/9
  From Spreadsheet/23 -> Vector Concatenate5/10
  From Spreadsheet/24 -> Vector Concatenate5/11
  From Spreadsheet/25 -> Vector Concatenate5/12
  From Spreadsheet/26 -> Vector Concatenate5/13
  From Spreadsheet/27 -> Vector Concatenate5/14
  From Spreadsheet/28 -> Vector Concatenate5/15
  From Spreadsheet/29 -> Vector Concatenate5/16
  From Spreadsheet/30 -> Vector Concatenate5/17
  From Spreadsheet/31 -> Vector Concatenate5/18
  Vector Concatenate/1 -> Gain1/1
  Data Type Conversion17/1 -> CurrentSense/1
  Vector Concatenate3/1 -> Temperatures1_C/1  "Temperatures1_C"
  Vector Concatenate4/1 -> Temperatures2_C/1  "Temperatures1_C"
  Vector Concatenate5/1 -> Data Type Conversion1/1
  From Spreadsheet/32 -> [dataFromTest]
  From Spreadsheet/33 -> [DCLO_test]
  connections:
  Battery8/LConn2 -- Voltage Measurement3/LConn2 -- Series RLC Branch9/RConn1 -- Ideal Switch4/LConn1 -- Voltage Measurement4/LConn1 -- Battery7/LConn1
  Series RLC Branch18/LConn1 -- Ideal Switch7/RConn1
  Voltage Measurement7/LConn2 -- Battery4/LConn2 -- Ideal Switch12/LConn1 -- Series RLC Branch24/RConn1 -- Voltage Measurement10/LConn1 -- Battery3/LConn1
  Voltage Measurement8/LConn1 -- Battery2/LConn1 -- Series RLC Branch33/RConn1 -- SBal0103/LConn1 -- Battery3/LConn2 -- Voltage Measurement10/LConn2
  RBal0101/LConn1 -- SBal0101/RConn1
  Voltage Measurement9/LConn1 -- Battery1/LConn1 -- SBal0102/LConn1 -- RBal0103/RConn1 -- Battery2/LConn2 -- Voltage Measurement8/LConn2
  Battery/LConn1 -- Voltage Measurement11/LConn1 -- SBal0101/LConn1 -- RBal0102/RConn1 -- Voltage Measurement9/LConn2 -- Battery1/LConn2
  Voltage Measurement12/LConn2 -- Battery12/LConn2 -- Ideal Switch/LConn1 -- Series RLC Branch1/RConn1 -- Battery11/LConn1 -- Voltage Measurement/LConn1
  Series RLC Branch7/RConn1 -- Voltage Measurement2/LConn1 -- Battery9/LConn1 -- Battery10/LConn2 -- Voltage Measurement1/LConn2 -- Ideal Switch2/LConn1
  Ideal Switch1/LConn1 -- Battery11/LConn2 -- Voltage Measurement/LConn2 -- Battery10/LConn1 -- Voltage Measurement1/LConn1 -- Series RLC Branch5/RConn1
  RBal0103/LConn1 -- SBal0103/RConn1
  Series RLC Branch7/LConn1 -- Ideal Switch1/RConn1
  RBal0102/LConn1 -- SBal0102/RConn1
  Series RLC Branch10/LConn1 -- Ideal Switch4/RConn1
  Series RLC Branch33/LConn1 -- Ideal Switch12/RConn1
  Series RLC Branch24/LConn1 -- Ideal Switch9/RConn1
  Series RLC Branch21/LConn1 -- Ideal Switch8/RConn1
  Battery5/LConn2 -- Voltage Measurement6/LConn2 -- Series RLC Branch21/RConn1 -- Ideal Switch9/LConn1 -- Battery4/LConn1 -- Voltage Measurement7/LConn1
  Battery7/LConn2 -- Ideal Switch7/LConn1 -- Series RLC Branch10/RConn1 -- Battery6/LConn1 -- Voltage Measurement5/LConn1 -- Voltage Measurement4/LConn2
  Series RLC Branch8/LConn1 -- Ideal Switch2/RConn1
  Voltage Measurement5/LConn2 -- Battery6/LConn2 -- Series RLC Branch18/RConn1 -- Ideal Switch8/LConn1 -- Voltage Measurement6/LConn1 -- Battery5/LConn1
  Ideal Switch/RConn1 -- Series RLC Branch5/LConn1
  Series RLC Branch9/LConn1 -- Ideal Switch3/RConn1
  Battery9/LConn2 -- Series RLC Branch8/RConn1 -- Ideal Switch3/LConn1 -- Battery8/LConn1 -- Voltage Measurement3/LConn1 -- Voltage Measurement2/LConn2
  Ideal Switch6/RConn1 -- Series RLC Branch1/LConn1
  Voltage Measurement13/LConn2 -- Battery13/LConn2 -- Ideal Switch6/LConn1 -- Series RLC Branch2/RConn1 -- Battery12/LConn1 -- Voltage Measurement12/LConn1
  Ideal Switch10/RConn1 -- Series RLC Branch2/LConn1
  Voltage Measurement14/LConn2 -- Battery14/LConn2 -- Ideal Switch10/LConn1 -- Series RLC Branch3/RConn1 -- Battery13/LConn1 -- Voltage Measurement13/LConn1
  Voltage Measurement15/LConn2 -- Battery15/LConn2 -- Ideal Switch11/LConn1 -- Series RLC Branch4/RConn1 -- Battery14/LConn1 -- Voltage Measurement14/LConn1
  Ideal Switch11/RConn1 -- Series RLC Branch3/LConn1
  Voltage Measurement16/LConn2 -- Battery16/LConn2 -- Ideal Switch13/LConn1 -- Series RLC Branch11/RConn1 -- Battery15/LConn1 -- Voltage Measurement15/LConn1
  Ideal Switch13/RConn1 -- Series RLC Branch4/LConn1
  Voltage Measurement17/LConn2 -- Battery17/LConn2 -- Ideal Switch14/LConn1 -- Series RLC Branch12/RConn1 -- Battery16/LConn1 -- Voltage Measurement16/LConn1
  Ideal Switch14/RConn1 -- Series RLC Branch11/LConn1
  Voltage Measurement18/LConn2 -- Battery18/LConn2 -- Ideal Switch15/LConn1 -- Series RLC Branch13/RConn1 -- Battery17/LConn1 -- Voltage Measurement17/LConn1
  Ideal Switch15/RConn1 -- Series RLC Branch12/LConn1
  Voltage Measurement19/LConn2 -- Battery19/LConn2 -- Ideal Switch16/LConn1 -- Series RLC Branch14/RConn1 -- Battery18/LConn1 -- Voltage Measurement18/LConn1
  Ideal Switch16/RConn1 -- Series RLC Branch13/LConn1
  Ideal Switch17/RConn1 -- Series RLC Branch14/LConn1
  Ideal Switch17/LConn1 -- Battery19/LConn1 -- Ideal Switch5/RConn1 -- Voltage Measurement19/LConn1
  RBal0101/RConn1 -- Controlled Current Source1/LConn1 -- Battery/LConn2 -- Voltage Measurement11/LConn2
  Current Measurement1/LConn1 -- Controlled Current Source1/RConn1
  Current Measurement1/RConn1 -- Ideal Switch5/LConn1
